simulink model "verify_CreateSdat_mdl"  (R2018b)
settings: Solver=VariableStepDiscrete  StartTime=0  StopTime=1  MaxStep=1  RelTol=1e-3  EnableMultiTasking=on
InitFcn:
  | load('DE_TRY2010_13_averageYear')
libraries: carnot x34
settings Model: Creator=drhf  LastModifiedBy=drhf
settings DataIOCC: SaveFormat=Array  SignalLoggingSaveFormat=ModelDataLogs
settings OptimizationCC: ExpressionDepthLimit=2147483647  LifeSpan=inf
settings DebuggingCC: UnderspecifiedInitializationDetection=Classic  MergeDetectMultiDrivingBlocksExec=none  SolverPrmCheckMsg=warning  FcnCallInpInsideContextMsg=warning  StateNameClashWarn=warning  SFUnexpectedBacktrackingDiag=warning  SFNoUnconditionalDefaultTransitionDiag=warning  SFExecutionAtInitializationDiag=none
settings HardwareCC: ProdBitPerPointer=32  ProdBitPerSizeT=32  ProdBitPerPtrDiffT=32  ProdLargestAtomicFloat=None  ProdIntDivRoundTo=Undefined  ProdEndianess=Unspecified  ProdWordSize=32  ProdHWDeviceType=32-bit Generic
settings ModelReferenceCC: PropagateSignalLabelsOutOfModel=off
settings SFSimCC: SimUseLocalCustomCode=off
settings RTWCC: RTWUseLocalCustomCode=off
settings CodeAppCC: StateflowObjectComments=on
settings GRTTargetCC: TargetLangStandard=C89/C90 (ANSI)  GeneratePreprocessorConditionals=Disable all  CombineOutputUpdateFcns=off  GRTInterface=on
settings ConfigComp: CovMetricSettings=dw  CovHtmlReporting=on  CovSaveCumulativeToWorkspaceVar=on  CovSaveSingleToWorkspaceVar=on  CovExternalEMLEnable=off

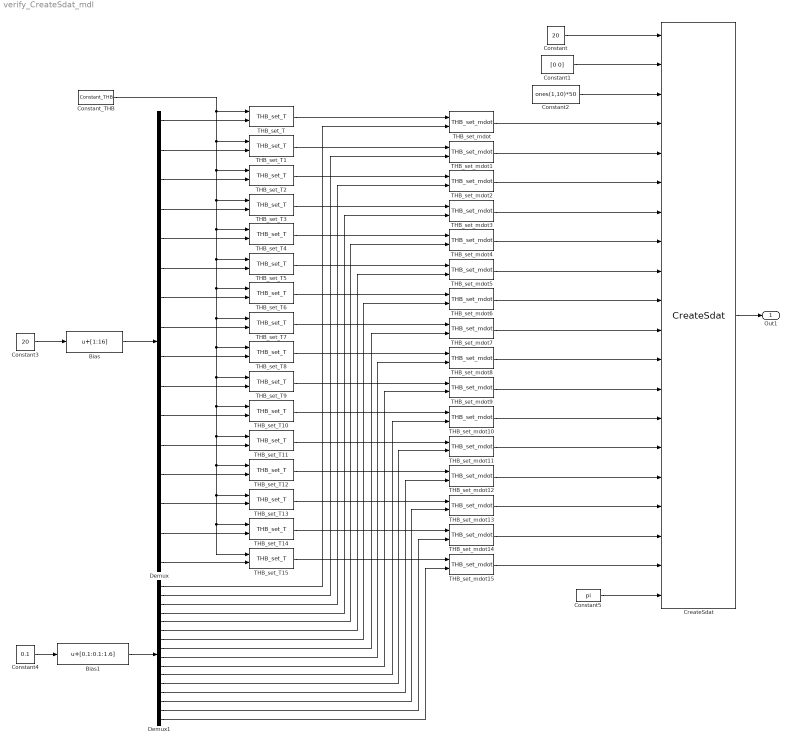
== system verify_CreateSdat_mdl ==
  Bias : Bias  Bias=[1:16]
  Bias1 : Bias  Bias=[0.1:0.1:1.6]
  Constant : Constant  Value=20
  Constant1 : Constant  Value=[0 0]
  Constant2 : Constant  Value=ones(1,10)*50
  Constant3 : Constant  Value=20
  Constant4 : Constant  Value=0.1
  Constant5 : Constant  Value=pi
  Constant_THB : carnot/Source/Simple/Constant_THB  t=20  mdot=0  p=1e5  mID=No Pressure Drop  fluid=Water  mix=0  mix2=0  mix3=0  dia=0.02  hgt=0
      settings: SourceProductName=Carnot
  CreateSdat : carnot/Basic/Thermal_Models/CreateSdat  volume=0.1  stgtype=1
      settings: SourceProductName=Carnot
  Demux : Demux  Outputs=16
  Demux1 : Demux  Outputs=16
  THB_set_T{,1..15} (16 alike) : carnot/Source/Simple/THB_set_T
      settings: SourceProductName=Carnot
  THB_set_mdot{,1..15} (16 alike) : carnot/Source/Simple/THB_set_mdot
      settings: SourceProductName=Carnot
  Out1 : Outport
  wires:
  CreateSdat/1 -> Out1/1
  Constant/1 -> CreateSdat/1
  Constant1/1 -> CreateSdat/2
  Constant2/1 -> CreateSdat/3
  Constant_THB/1 -> THB_set_T2/1, THB_set_T4/1, THB_set_T5/1, THB_set_T6/1, THB_set_T8/1, THB_set_T9/1, THB_set_T10/1, THB_set_T11/1, THB_set_T12/1, THB_set_T13/1, THB_set_T14/1, THB_set_T15/1, THB_set_T7/1, THB_set_T3/1, THB_set_T1/1, THB_set_T/1
  THB_set_T/1 -> THB_set_mdot/1
  THB_set_mdot/1 -> CreateSdat/4
  Constant3/1 -> Bias/1
  THB_set_T1/1 -> THB_set_mdot1/1
  THB_set_T2/1 -> THB_set_mdot2/1
  THB_set_T3/1 -> THB_set_mdot3/1
  THB_set_T4/1 -> THB_set_mdot4/1
  THB_set_T5/1 -> THB_set_mdot5/1
  THB_set_T6/1 -> THB_set_mdot6/1
  THB_set_T7/1 -> THB_set_mdot7/1
  Bias/1 -> Demux/1
  Demux/1 -> THB_set_T/2
  Demux/2 -> THB_set_T1/2
  Demux/3 -> THB_set_T2/2
  Demux/4 -> THB_set_T3/2
  Constant4/1 -> Bias1/1
  Bias1/1 -> Demux1/1
  Demux/5 -> THB_set_T4/2
  Demux1/1 -> THB_set_mdot/2
  Demux1/2 -> THB_set_mdot1/2
  THB_set_mdot1/1 -> CreateSdat/5
  THB_set_mdot2/1 -> CreateSdat/6
  THB_set_mdot3/1 -> CreateSdat/7
  THB_set_mdot4/1 -> CreateSdat/8
  THB_set_mdot5/1 -> CreateSdat/9
  THB_set_mdot6/1 -> CreateSdat/10
  THB_set_mdot7/1 -> CreateSdat/11
  Demux/6 -> THB_set_T5/2
  Demux/7 -> THB_set_T6/2
  Demux/8 -> THB_set_T7/2
  Demux1/3 -> THB_set_mdot2/2
  Demux1/8 -> THB_set_mdot7/2
  Demux1/7 -> THB_set_mdot6/2
  Demux1/6 -> THB_set_mdot5/2
  Demux1/5 -> THB_set_mdot4/2
  Demux1/4 -> THB_set_mdot3/2
  THB_set_T15/1 -> THB_set_mdot15/1
  THB_set_T14/1 -> THB_set_mdot14/1
  THB_set_T13/1 -> THB_set_mdot13/1
  THB_set_T12/1 -> THB_set_mdot12/1
  THB_set_T11/1 -> THB_set_mdot11/1
  THB_set_T10/1 -> THB_set_mdot10/1
  THB_set_T9/1 -> THB_set_mdot9/1
  THB_set_T8/1 -> THB_set_mdot8/1
  THB_set_mdot8/1 -> CreateSdat/12
  THB_set_mdot9/1 -> CreateSdat/13
  THB_set_mdot10/1 -> CreateSdat/14
  THB_set_mdot11/1 -> CreateSdat/15
  THB_set_mdot12/1 -> CreateSdat/16
  THB_set_mdot13/1 -> CreateSdat/17
  THB_set_mdot14/1 -> CreateSdat/18
  THB_set_mdot15/1 -> CreateSdat/19
  Constant5/1 -> CreateSdat/20
  Demux/16 -> THB_set_T15/2
  Demux/9 -> THB_set_T8/2
  Demux/10 -> THB_set_T9/2
  Demux/11 -> THB_set_T10/2
  Demux/12 -> THB_set_T11/2
  Demux/13 -> THB_set_T12/2
  Demux/14 -> THB_set_T13/2
  Demux/15 -> THB_set_T14/2
  Demux1/9 -> THB_set_mdot8/2
  Demux1/10 -> THB_set_mdot9/2
  Demux1/11 -> THB_set_mdot10/2
  Demux1/12 -> THB_set_mdot11/2
  Demux1/13 -> THB_set_mdot12/2
  Demux1/14 -> THB_set_mdot13/2
  Demux1/15 -> THB_set_mdot14/2
  Demux1/16 -> THB_set_mdot15/2
